simulink model "QP_solver"  (R2020b)
settings: Solver=FixedStepAuto  StartTime=0.0  StopTime=15  FixedStep=1/400  RelTol=1e-3
settings Model: Creator=86152  LastModifiedBy=86152
settings OptimizationCC: DefaultParameterBehavior=Inlined  UseDivisionForNetSlopeComputation=on  GainParamInheritBuiltInType=on  UseFloatMulNetSlope=on  InlineInvariantSignals=on  EnhancedBackFolding=on  PassReuseOutputArgsAs=Individual arguments  ZeroExternalMemoryAtStartup=off  ZeroInternalMemoryAtStartup=off  EfficientFloat2IntCast=on  OptimizeBlockOrder=speed  DifferentSizesBufferReuse=on  OptimizationCustomize=off  EfficientTunableParamExpr=on
settings DebuggingCC: ParameterTunabilityLossMsg=error  SFUnexpectedBacktrackingDiag=warning  SFNoUnconditionalDefaultTransitionDiag=warning
settings HardwareCC: ProdLongLongMode=on
settings SFSimCC: MATLABDynamicMemAlloc=off
settings RTWCC: Description=Embedded Coder  SystemTargetFile=ert.tlc  GenCodeOnly=on  PackageGeneratedCodeAndArtifacts=on  PackageName=QP_solver.zip  TemplateMakefile=ert_default_tmf  GenerateReport=on  BuildConfiguration=Faster Runs  LaunchReport=on
settings CodeAppCC: ForceParamTrailComments=on  IgnoreCustomStorageClasses=off  OperatorAnnotations=on  SimulinkDataObjDesc=on  SFDataObjDesc=on  InsertBlockDesc=on  EnableCustomComments=on
settings ERTTargetCC: TargetLangStandard=C99 (ISO)  GenerateSampleERTMain=on  InlinedParameterPlacement=NonHierarchical  ERTCustomFileTemplate=example_file_process.tlc

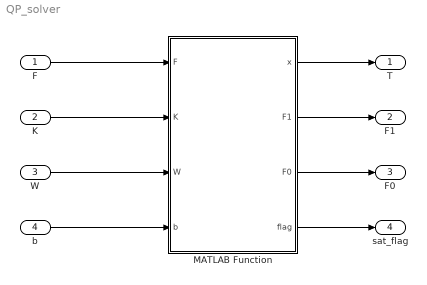
== system QP_solver ==
  F : Inport  PortDimensions=[4,1]
  K : Inport  Port=2  PortDimensions=[4,4]
  W : Inport  Port=3  PortDimensions=[4,1]
  b : Inport  Port=4  PortDimensions=[4,1]
  MATLAB Function : MATLAB Function  TreatAsAtomicUnit=on
  T : Outport
  F1 : Outport  Port=2
  F0 : Outport  Port=3
  sat_flag : Outport  Port=4
  wires:
  F/1 -> MATLAB Function/1(F)
  MATLAB Function/1(x) -> T/1
  MATLAB Function/2(F1) -> F1/1
  MATLAB Function/3(F0) -> F0/1
  MATLAB Function/4(flag) -> sat_flag/1
  W/1 -> MATLAB Function/3(W)
  b/1 -> MATLAB Function/4(b)
  K/1 -> MATLAB Function/2(K)

== matlab function QP_solver/MATLAB Function ==
  data: F input; K input; x output; W input; b input; F1 output; F0 output; flag output
function [x, F1, F0, flag] = mixer_solver(F, K, W, b)
if sum(sum(K)) < 0.001
    K = [-0.25 0.25 0.25 -0.25;
         0.25 0.25 -0.25 -0.25;
         0.25 -0.25 0.25 -0.25;
         0.25 0.25 0.25 0.25];
end
if sum(W) < 0.001
    W = diag([1 1 1 1]);
else
    W = diag(W);
end

lb = b(1) * ones(4,1);
ub = b(2) * ones(4,1);

F0 = F;
P = 2 * K' * W * K;
q = (-2 * K' * W * F);

opts = optimoptions('quadprog','Algorithm','active-set');
x0 = [0;0;0;0];
x = quadprog(P,q,[],[],[],[],lb,ub,x0,opts);
F1 = K * x;

if norm(F - F1) > 0.001
    flag = 1;
else
    flag = 0;
end
